simulink subsystem "observador_discreto"  (R2023b)
settings: Solver=VariableStepAuto  StartTime=0.0  StopTime=10.0  RelTol=1e-3
values from neighbouring files (symbols this model uses):
  J_eq = 1.9785e-5    (= 1.9785e-05)    [diagrama_polos_y_ceros_LTI.m]    (also in main.m = 1.97847222222e-05; parametros.m = 1.97847222222e-05)
undefined symbols (not defined in the file or in its folder): kem_i, kem_theta, kem_w
settings Model: Creator=nicol  LastModifiedBy=nicol

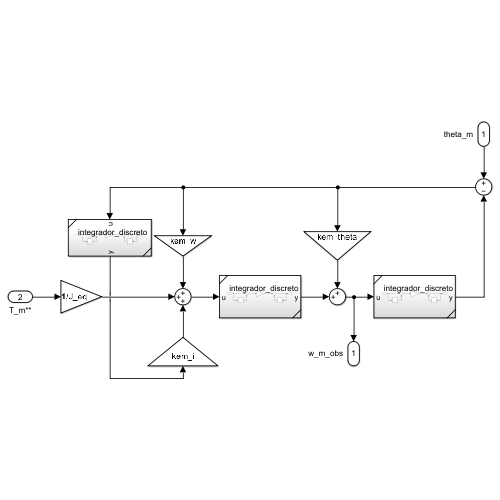
[thumbnail: Simulink's stored preview of the top-level diagram]
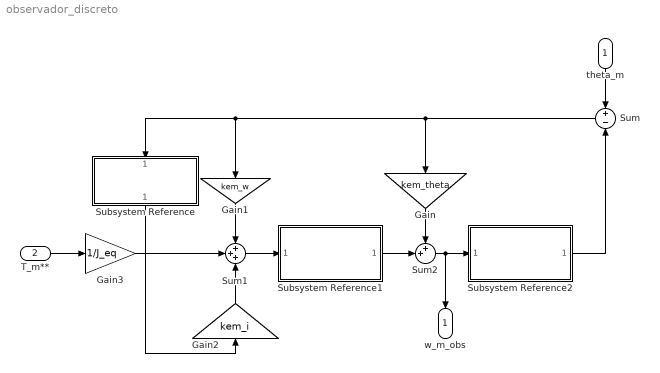
== system observador_discreto ==
  theta_m : Inport
  T_m** : Inport  Port=2
  Gain : Gain  Gain=kem_theta
  Gain1 : Gain  Gain=kem_w
  Gain2 : Gain  Gain=kem_i
  Gain3 : Gain  Gain=1/J_eq
  Subsystem Reference : Subsystem  ReferencedSubsystem=integrador_discreto
  Subsystem Reference1 : Subsystem  ReferencedSubsystem=integrador_discreto
  Subsystem Reference2 : Subsystem  ReferencedSubsystem=integrador_discreto
  Sum : Sum  Inputs=+-
  Sum1 : Sum  Inputs=+++
  Sum2 : Sum  Inputs=++|
  w_m_obs : Outport
  wires:
  Subsystem Reference2/1 -> Sum/2
  Sum1/1 -> Subsystem Reference1/1
  Subsystem Reference1/1 -> Sum2/2
  theta_m/1 -> Sum/1
  Gain2/1 -> Sum1/3
  Gain/1 -> Sum2/1
  Sum2/1 -> Subsystem Reference2/1, w_m_obs/1
  Subsystem Reference/1 -> Gain2/1
  T_m**/1 -> Gain3/1
  Sum/1 -> Gain/1, Subsystem Reference/1, Gain1/1
  Gain3/1 -> Sum1/2
  Gain1/1 -> Sum1/1
